simulink model "KNN"  (R2024b)
settings: Solver=VariableStepAuto  StartTime=0.0  StopTime=20  RelTol=1e-3
settings Model: Creator=Aleksandar  LastModifiedBy=Aleksandar

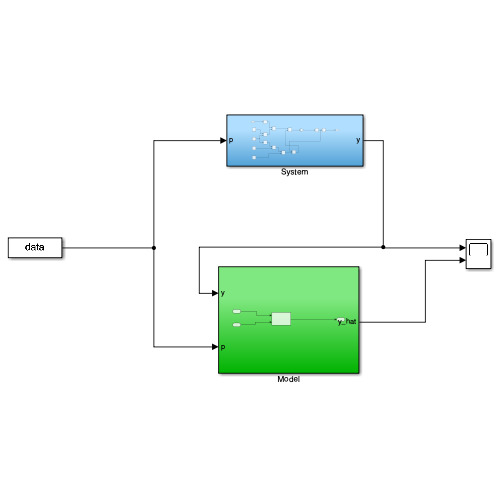
[thumbnail: Simulink's stored preview of the top-level diagram]
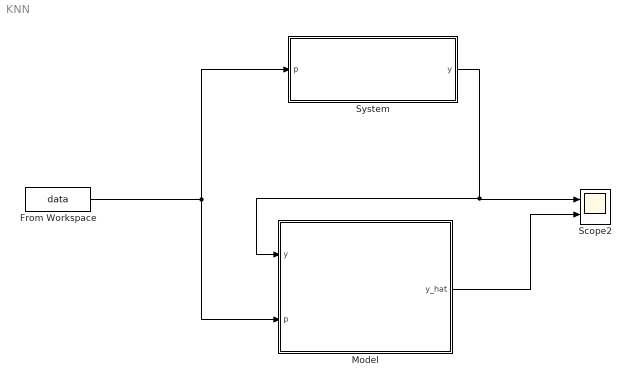
== system KNN ==
  From Workspace : FromWorkspace  VariableName=data  OutDataTypeStr=double  SampleTime=-1
  Model : Subsystem
  Scope2 : Scope  NumInputPorts=2
  System : Subsystem
  wires:
  System/1(y) -> Scope2/1, Model/1(y)
  From Workspace/1 -> Model/2(p), System/1(p)
  Model/1(y_hat) -> Scope2/2

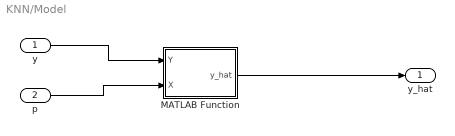
== system KNN/Model ==
  y : Inport
  p : Inport  Port=2
  MATLAB Function : MATLAB Function  TreatAsAtomicUnit=on
  y_hat : Outport
  wires:
  y/1 -> MATLAB Function/1(Y)
  p/1 -> MATLAB Function/2(X)
  MATLAB Function/1(y_hat) -> y_hat/1

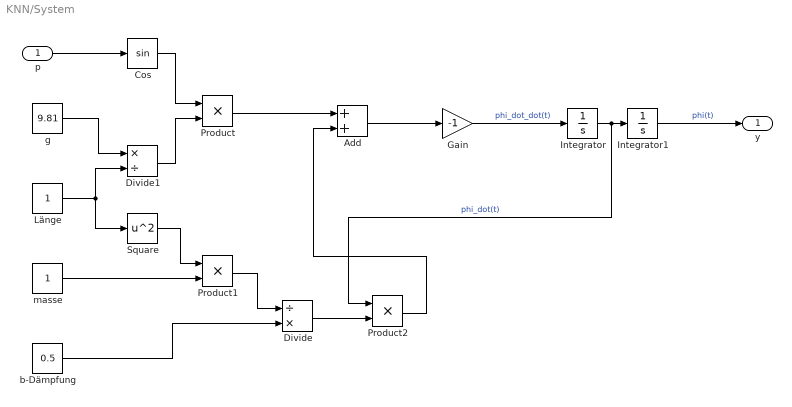
== system KNN/System ==
  p : Inport
  Add : Sum
  Cos : Trigonometry
  Divide : Product  Inputs=/*
  Divide1 : Product  Inputs=*/
  Gain : Gain  Gain=-1
  Integrator : Integrator
  Integrator1 : Integrator  InitialCondition=1.5708
  Länge : Constant
  Product : Product
  Product1 : Product
  Product2 : Product
  Square : Math  Operator=square
  b-Dämpfung : Constant  Value=0.5
  g : Constant  Value=9.81
  masse : Constant
  y : Outport
  wires:
  Integrator/1 -> Product2/1, Integrator1/1  "phi_dot(t)"
  Länge/1 -> Square/1, Divide1/2
  g/1 -> Divide1/1
  Integrator1/1 -> y/1  "phi(t)"
  Divide/1 -> Product2/2
  Cos/1 -> Product/1
  Product2/1 -> Add/2
  Product1/1 -> Divide/1
  b-Dämpfung/1 -> Divide/2
  Gain/1 -> Integrator/1  "phi_dot_dot(t)"
  Square/1 -> Product1/1
  Product/1 -> Add/1
  Divide1/1 -> Product/2
  masse/1 -> Product1/2
  Add/1 -> Gain/1
  p/1 -> Cos/1

== matlab function KNN/Model/MATLAB Function ==
  settings: updateMethod=DISCRETE
  data: Y input; y_hat output; X input
function y_hat = fcn(Y,X)
    
    i = 1;

    inputSize = 1; % Anzahl der Eingabeneuronen
    hiddenSize = 3; % Anzahl der Neuronen in der versteckten Schicht
    outputSize = 1; % Anzahl der Ausgabeneuronen
    
    % Zufällige Gewichte und Biases initialisieren
    W1 = rand(inputSize, hiddenSize); % Gewichte von Eingabe zu versteckter Schicht
    b1 = rand(1, hiddenSize); % Biases für versteckte Schicht
    W2 = rand(hiddenSize, outputSize); % Gewichte von versteckter zu Ausgabeschicht
    b2 = rand(1, outputSize); % Biases für Ausgabeschicht
    
    % Lernrate
    learningRate = 0.01;
    
    % Array zur Speicherung der Verlustwerte
    loss_values = zeros(1,100);

    % Anzahl der Epochen
    epochs = 1000;
    
    % Training des MLP
    for epoch = 1:epochs
        % Vorwärtsdurchlauf
        % Versteckte Schicht
        Z1 = X * W1 + b1; % Lineare Kombination
        A1 = tanh(Z1); % Aktivierungsfunktion (Tanh)
    
        % Ausgabeschicht
        Z2 = A1 * W2 + b2; % Lineare Kombination (keine Aktivierungsfunktion)
    
        % Verlustfunktion (Mean Squared Error)
        loss = mean(sum((Z2 - Y).^2, 2));
    
        % Rückpropagation
        % Fehler im Ausgabelayer
        dZ2 = Z2 - Y;
        dW2 = (A1' * dZ2) / size(X, 1);
        db2 = sum(dZ2, 1) / size(X, 1);
    
        % Fehler im versteckten Layer
        dA1 = dZ2 * W2';
        dZ1 = dA1 .* tanh_derivative(Z1);
        dW1 = (X' * dZ1) / size(X, 1);
        db1 = sum(dZ1, 1) / size(X, 1);
    
        % Parameteraktualisierung
        W1 = W1 - learningRate * dW1;
        b1 = b1 - learningRate * db1;
        W2 = W2 - learningRate * dW2;
        b2 = b2 - learningRate * db2;

        % Verlustwert alle 10 Epochen speichern
        if mod(epoch, 10) == 0
            loss_values(i) = loss;
            i = i+1;
        end
    
        % Ausgabe des Verlusts alle 100 Epochen
        if mod(epoch, 100) == 0
        %    fprintf('Epoch %d, Loss: %.4f\n', epoch, loss);
        end
    end
    
    % Ausgabe des trainierten MLP
    disp('Trainiertes MLP:');
    disp(Z2);
    
    % Verlustfunktion plotten
    figure;
    plot(loss_values, '-o');
    xlabel('Epoch');
    ylabel('Loss');
    title('Loss Function over Epochs');
    
    % Tanh-Aktivierungsfunktion
    function y = tanh(x)
        y = (exp(x) - exp(-x)) ./ (exp(x) + exp(-x));
    end
    
    % Ableitung der Tanh-Aktivierungsfunktion
    function y = tanh_derivative(x)
        y = 1 - tanh(x).^2;
    end


y_hat = Z2;

end
